simulink model "Models"  (R2020a)
settings: Solver=VariableStepAuto  StartTime=0.0  StopTime=30  RelTol=1e-3
settings Model: Creator=hussein  LastModifiedBy=hussein

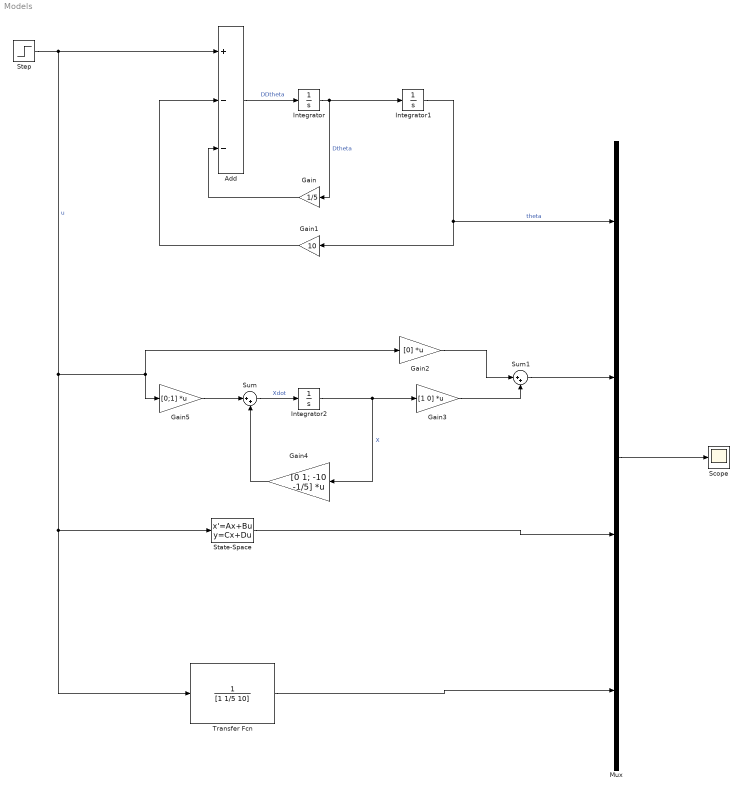
== system Models ==
  Add : Sum  Inputs=+--
  Gain : Gain  Gain=1/5
  Gain1 : Gain  Gain=10
  Gain2 : Gain  Gain=[0]  Multiplication=Matrix(K*u)
  Gain3 : Gain  Gain=[1 0]  Multiplication=Matrix(K*u)
  Gain4 : Gain  Gain=[0 1; -10 -1/5]  Multiplication=Matrix(K*u)
  Gain5 : Gain  Gain=[0;1]  Multiplication=Matrix(K*u)
  Integrator : Integrator
  Integrator1 : Integrator
  Integrator2 : Integrator
  Mux : Mux
  Scope : Scope
  State-Space : StateSpace  A=[0 1; -10 -1/5]  B=[0;1]  C=[1 0]  D=[0]  InitialCondition=0
  Step : Step  Time=3  SampleTime=0
  Sum : Sum  Inputs=|++
  Sum1 : Sum  Inputs=|++
  Transfer Fcn : TransferFcn  Denominator=[1 1/5 10]
  wires:
  Step/1 -> State-Space/1, Transfer Fcn/1, Gain5/1, Gain2/1, Add/1  "u"
  Add/1 -> Integrator/1  "DDtheta"
  Integrator/1 -> Gain/1, Integrator1/1  "Dtheta"
  Gain/1 -> Add/3
  Integrator1/1 -> Gain1/1, Mux/1  "theta"
  Gain1/1 -> Add/2
  Sum/1 -> Integrator2/1  "Xdot"
  Gain4/1 -> Sum/2
  Gain3/1 -> Sum1/2
  Integrator2/1 -> Gain4/1, Gain3/1  "X"
  Gain2/1 -> Sum1/1
  Gain5/1 -> Sum/1
  Sum1/1 -> Mux/2
  Mux/1 -> Scope/1
  State-Space/1 -> Mux/3
  Transfer Fcn/1 -> Mux/4
